simulink model "batchTestIntakeIsothermal"  (R2024b)
settings: Solver=ode23t  StartTime=0.0  StopTime=3.0  MaxStep=0.1  RelTol=1e-3
libraries: nesl_utility x6, engine_lib x1
settings Model: SimulationMode=accelerator  Creator=264629  LastModifiedBy=isaacito
settings SolverCC: AlgebraicLoopSolver=TrustRegion
settings DataIOCC: SaveOutput=off  DSMLogging=off  SaveTime=off  ReturnWorkspaceOutputs=off  SignalLoggingName=loggedSignals  OutputOption=SpecifiedOutputTimes  OutputTimes=[2 3]
settings OptimizationCC: EfficientMapNaN2IntZero=off
settings DebuggingCC: UnconnectedInputMsg=warning  UnconnectedOutputMsg=warning  UnconnectedLineMsg=warning  ArithmeticOperatorsInVariantConditions=warning
settings HardwareCC: TargetBitPerPointer=64  TargetBitPerSizeT=64  TargetBitPerPtrDiffT=64  TargetLongLongMode=on  TargetIntDivRoundTo=Zero  TargetEndianess=LittleEndian  TargetWordSize=64  TargetHWDeviceType=MATLAB Host  ProdEqTarget=off
settings ModelReferenceCC: EnableRefExpFcnMdlSchedulingChecks=on
settings SFSimCC: SimUseLocalCustomCode=off  CustomCodeUndefinedFunction=UseInterfaceOnly
settings RTWCC: RTWUseLocalCustomCode=off  GPUComputeCapability=3.5
settings CodeAppCC: MaxIdLength=128
settings GRTTargetCC: TargetLangStandard=C89/C90 (ANSI)  CombineOutputUpdateFcns=off  GRTInterface=on
settings SimscapeCC: SimscapeNormalizeSystem=off  SimscapeLogSimulationStatistics=on  SimscapeLogLimitData=off

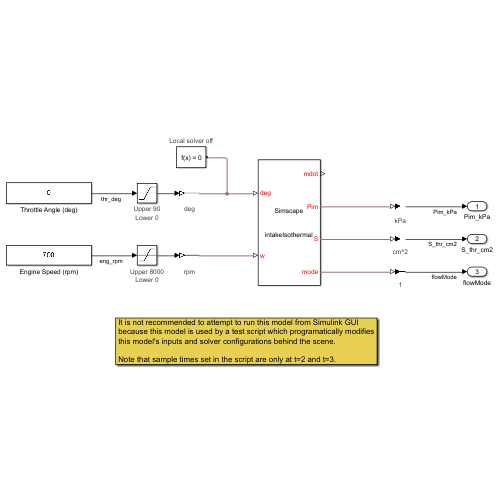
[thumbnail: Simulink's stored preview of the top-level diagram]
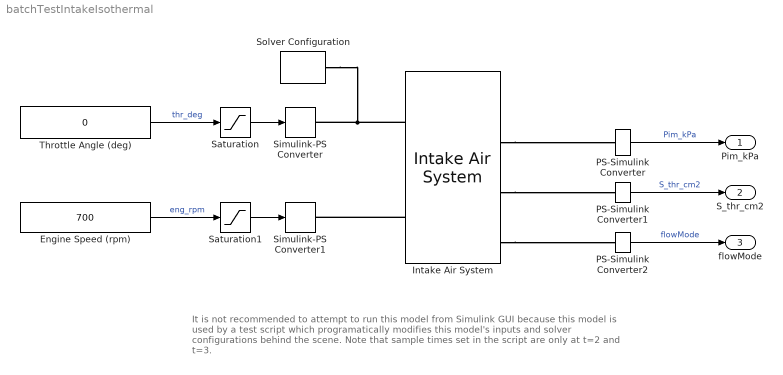
== system batchTestIntakeIsothermal ==
  note: It is not recommended to attempt to run this model from Simulink GUI
      | because this model is used by a test script which programatically modifies
      | this model's inputs and solver configurations behind the scene.
      |
      | Note that sample times set in the script are only at t=2 and t=3.
  Engine Speed (rpm) : Constant  Value=700
  Intake Air System : engine_lib/Intake Air System
      settings: InternalSimscapePortConfiguration="{\"Bottom\":[],\"Left\":[{\"id\":\"thr_cmd\",\"label\":\"deg\",\"type\":\"input\"},{\"id\":\"w\",\"label\":\"w\",\"type\":\"input\"}],\"Right\":[{\"id\":\"mdot_tocyl\",\"label\":\"mdot\",\"type\":\"output\"},{\"id\":\"p_im_out\",\"label\":\"Pim\",\"type\":\"output\"},{\"id\":\"S_thr\",\"label\":\"S\",\"type\":\"output\"},{\"id\":\"flowMode\",\"label\":\"mode\",\"type\":\"output\"}],\"Top\":[]}"
  PS-Simulink Converter : nesl_utility/PS-Simulink Converter  PhysicalDomain=network_engine_domain  SubClassName=ps_output  LeftPortType=input  RightPortType=output  PseudoPeriodic=off  Frequencies=[]  VectorFormat=1-D array  Unit=kPa  AffineConversion=off
  PS-Simulink Converter1 : nesl_utility/PS-Simulink Converter  PhysicalDomain=network_engine_domain  SubClassName=ps_output  LeftPortType=input  RightPortType=output  PseudoPeriodic=off  Frequencies=[]  VectorFormat=1-D array  Unit=cm^2  AffineConversion=off
  PS-Simulink Converter2 : nesl_utility/PS-Simulink Converter  PhysicalDomain=network_engine_domain  SubClassName=ps_output  LeftPortType=input  RightPortType=output  PseudoPeriodic=off  Frequencies=[]  VectorFormat=1-D array  Unit=1  AffineConversion=off
  Saturation : Saturate  UpperLimit=90  LowerLimit=0
      settings: AttributesFormatString=|
      | Upper %<UpperLimit>
      | Lower %<LowerLimit>
  Saturation1 : Saturate  UpperLimit=8000  LowerLimit=0
      settings: AttributesFormatString=|
      | Upper %<UpperLimit>
      | Lower %<LowerLimit>
  Simulink-PS Converter : nesl_utility/Simulink-PS Converter  PhysicalDomain=network_engine_domain  SubClassName=ps_input  LeftPortType=input  RightPortType=output  PseudoPeriodic=off  Frequencies=[]  NoiseDistribution=none  NoiseParameters=[]  Unit=deg  AffineConversion=off  FilteringAndDerivatives=provide  SimscapeFilterOrder=1  InputFilterTimeConstant=0.001  UdotUserProvided=0
  Simulink-PS Converter1 : nesl_utility/Simulink-PS Converter  PhysicalDomain=network_engine_domain  SubClassName=ps_input  LeftPortType=input  RightPortType=output  PseudoPeriodic=off  Frequencies=[]  NoiseDistribution=none  NoiseParameters=[]  Unit=rpm  AffineConversion=off  FilteringAndDerivatives=provide  SimscapeFilterOrder=1  InputFilterTimeConstant=0.001  UdotUserProvided=0
  Solver Configuration : nesl_utility/Solver Configuration  PhysicalDomain=network_engine_domain  SubClassName=solver  LeftPortType=input  RightPortType=generic  Tones=[]  Harmonics=[]  SimulateNoise=off  Profile=off  UseLocalSampling=off  EnableSwitchedLinearOptims=on  FrequencyDomain=off  UseCCode=off  RelTol=0.001  AbsTol=1e-06  MinStep=1e-09  ToWorkspace=off  RevertToSquareIcSolve=off  NumHomotopyIterations=100  PhasorMode=off  PhasorModeNumHarmonics=1  ConsistencySolver=NEWTON_FTOL  IndexReductionMethod=DerivativeReplacement  DoDC=off  ResidualTolerance=1e-09  ConsistencyTolSource=GLOBAL  ConsistencyAbsTol=0.001  ConsistencyRelTol=0.001  ConsistencyTolFactor=0.001  UseLocalSolver=off  LocalSolverChoice=NE_BACKWARD_EULER_ADVANCER  ResolveIndetEquations=on  FunctionEvalNumThread=1  LocalSolverSampleTime=0.001  DoFixedCost=off  MaxNonlinIter=3  MaxModeIter=2  ComputeImpulses=off  ImpulseIterations=2  LinearAlgebra=Sparse  LinearAlgebraNumThread=0  EquationFormulation=NE_TIME_EF  DelaysMemoryBudget=1024  AutomaticFiltering=on  FilteringTimeConstant=0.001  PartitionStorageMethod=AS_NEEDED  PartitionMemoryBudget=1024  PartitionMethod=FAST  MultibodyUseLocalSolver=off  MultibodyLocalSolverChoice=ODE1  MultibodyLocalSolverSampleTime=0.001
      settings: AttributesFormatString=Local solver %<UseLocalSolver>
  Throttle Angle (deg) : Constant  Value=0
  Pim_kPa : Outport  VectorParamsAs1DForOutWhenUnconnected=off
  S_thr_cm2 : Outport  Port=2  VectorParamsAs1DForOutWhenUnconnected=off
  flowMode : Outport  Port=3  VectorParamsAs1DForOutWhenUnconnected=off
  wires:
  Throttle Angle (deg)/1 -> Saturation/1  "thr_deg"
  Engine Speed (rpm)/1 -> Saturation1/1  "eng_rpm"
  PS-Simulink Converter/1 -> Pim_kPa/1  "Pim_kPa"
  Saturation/1 -> Simulink-PS Converter/1
  Saturation1/1 -> Simulink-PS Converter1/1
  PS-Simulink Converter1/1 -> S_thr_cm2/1  "S_thr_cm2"
  PS-Simulink Converter2/1 -> flowMode/1  "flowMode"
  connections:
  Solver Configuration/RConn1 -- Intake Air System/LConn1 -- Simulink-PS Converter/RConn1
  Intake Air System/LConn2 -- Simulink-PS Converter1/RConn1
  Intake Air System/RConn4 -- PS-Simulink Converter2/LConn1
  Intake Air System/RConn3 -- PS-Simulink Converter1/LConn1
  Intake Air System/RConn2 -- PS-Simulink Converter/LConn1
